simulink model "main_ddp_N5"  (R2026a)
settings: Solver=VariableStepAuto  StopTime=simulation_time  FixedStep=params.MPC.dt  RelTol=1e-2
undefined symbols (not defined in the file or in its folder): params, Ref
(part 1 of 2)
settings Model: Creator=katsu  LastModifiedBy=hoshino

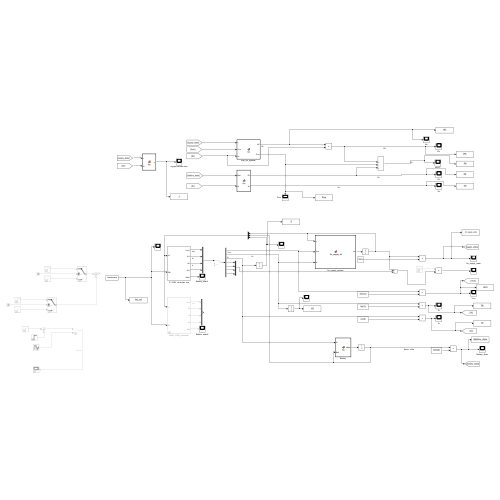
[thumbnail: Simulink's stored preview of the top-level diagram]
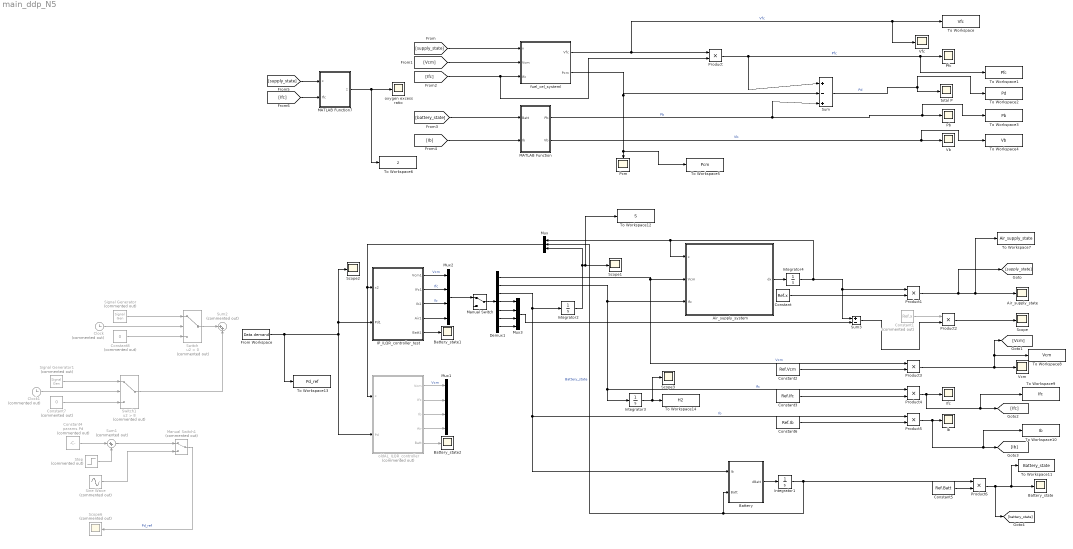
== system main_ddp_N5 ==
  Air_supply_state : Scope
      settings: ActiveDisplayYMinimum=-12592.967592784222  ActiveDisplayYMaximum=162770.79990525215  DataLoggingVariableName=ScopeData3
  Air_supply_system : MATLAB Function  TreatAsAtomicUnit=on
  Battery : MATLAB Function  TreatAsAtomicUnit=on
  Battery_state : Scope
      settings: ActiveDisplayYMinimum=-1  ActiveDisplayYMaximum=1  DataLoggingVariableName=ScopeData2
  Battery_state1 : Scope
      settings: ActiveDisplayYMinimum=-0.0625  ActiveDisplayYMaximum=0.5625
  Battery_state2 : Scope
      settings: ActiveDisplayYMinimum=-0.0625  ActiveDisplayYMaximum=0.5625
  Clock : Clock  Commented=on
  Clock1 : Clock  Commented=on
  Constant : Constant  Value=Ref.x
  Constant1 : Constant  Commented=on  Value=Ref.x
  Constant2 : Constant  Value=Ref.Vcm
  Constant3 : Constant  Value=Ref.Ifc
  Constant4 : Constant  Commented=on  Value=params.Pd
  Constant5 : Constant  Value=Ref.Batt
  Constant6 : Constant  Value=Ref.Ib
  Constant7 : Constant  Commented=on  Value=0
  Constant8 : Constant  Commented=on  Value=0
  Demux1 : Demux  Outputs=7
  From Workspace : FromWorkspace  VariableName=Data.demand
  IP_ILQR_controller_test : Subsystem
  Ib : Scope
      settings: ActiveDisplayYMinimum=-4.4974516854867295  ActiveDisplayYMaximum=40.486661709078128  DataLoggingVariableName=ScopeData3
  Ifc : Scope
      settings: ActiveDisplayYMinimum=31.92108  ActiveDisplayYMaximum=418.48985  DataLoggingVariableName=ScopeData2
  Integrator1 : Integrator  InitialCondition=params.start.Bat./Ref.Batt
  Integrator2 : Integrator
  Integrator3 : Integrator
  Integrator4 : Integrator  InitialCondition=params.start.x ./[Ref.x]
  MATLAB Function : MATLAB Function  TreatAsAtomicUnit=on
  MATLAB Function7 : MATLAB Function  TreatAsAtomicUnit=on
  Manual Switch : ManualSwitch
  Manual Switch1 : ManualSwitch  Commented=on
  Mux : Mux  Inputs=3
  Mux1 : Mux
  Mux2 : Mux
  Mux3 : Mux
  Pb : Scope
      settings: ActiveDisplayYMinimum=-1  ActiveDisplayYMaximum=1  DataLoggingVariableName=ScopeData6
  Pcm : Scope
      settings: ActiveDisplayYMinimum=1718.35704  ActiveDisplayYMaximum=9747.00989  DataLoggingVariableName=ScopeData4
  Pfc : Scope
      settings: ActiveDisplayYMinimum=-1238.1930512276633  ActiveDisplayYMaximum=24168.684595902479  DataLoggingVariableName=ScopeData5
  Product{,1..6} (7 alike) : Product
  Scope{,1..3} (4 alike) : Scope
      Scope settings: ActiveDisplayYMinimum=-1  ActiveDisplayYMaximum=1  DataLoggingVariableName=ScopeData3
      Scope1 settings: ActiveDisplayYMinimum=-0.37216  ActiveDisplayYMaximum=2.27993
      Scope2 settings: ActiveDisplayYMinimum=20919.76712  ActiveDisplayYMaximum=45919.76712
      Scope3 settings: ActiveDisplayYMinimum=-0.23032  ActiveDisplayYMaximum=2.07287
  Scope6 : Scope  Commented=on
      settings: ActiveDisplayYMinimum=23419.76712  ActiveDisplayYMaximum=33419.76712
  Signal Generator : SignalGenerator  Commented=on  WaveForm=square  Amplitude=10000  Frequency=0.5  Units=rad/sec
  Signal Generator1 : SignalGenerator  Commented=on  WaveForm=square  Amplitude=10000  Frequency=0.8  Units=rad/sec
  Sine Wave : Sin  Commented=on  Amplitude=1000  Bias=params.Pd  SampleTime=0
  Step : Step  Commented=on  FinalValue=10000  SampleTime=0
  Sum : Sum  Inputs=|+-+
  Sum1 : Sum  Commented=on  Inputs=|++
  Sum2 : Sum  Commented=on  Inputs=|++
  Sum3 : Sum  Inputs=+-
  Switch : Switch  Commented=on  Criteria=u2 > Threshold  SaturateOnIntegerOverflow=off  InputSameDT=off
  Switch1 : Switch  Commented=on  Criteria=u2 > Threshold  Threshold=8  SaturateOnIntegerOverflow=off  InputSameDT=off
  To Workspace : ToWorkspace  VariableName=Vfc  SaveFormat=Timeseries  SampleTime=-1
  To Workspace1 : ToWorkspace  VariableName=Pfc  SaveFormat=Timeseries  SampleTime=-1
  To Workspace10 : ToWorkspace  VariableName=Ib  SaveFormat=Timeseries  SampleTime=-1
  To Workspace11 : ToWorkspace  VariableName=Battery_state  SaveFormat=Timeseries  SampleTime=-1
  To Workspace12 : ToWorkspace  VariableName=S  SaveFormat=Timeseries  SampleTime=-1
  To Workspace13 : ToWorkspace  VariableName=Pd_ref  SaveFormat=Timeseries  SampleTime=-1
  To Workspace14 : ToWorkspace  VariableName=H2  SaveFormat=Timeseries  SampleTime=-1
  To Workspace2 : ToWorkspace  VariableName=Pd  SaveFormat=Timeseries  SampleTime=-1
  To Workspace3 : ToWorkspace  VariableName=Pb  SaveFormat=Timeseries  SampleTime=-1
  To Workspace4 : ToWorkspace  VariableName=Vb  SaveFormat=Timeseries  SampleTime=-1
  To Workspace5 : ToWorkspace  VariableName=Pcm  SaveFormat=Timeseries  SampleTime=-1
  To Workspace6 : ToWorkspace  VariableName=z  SaveFormat=Timeseries  SampleTime=-1
  To Workspace7 : ToWorkspace  VariableName=Air_supply_state  SaveFormat=Timeseries  SampleTime=-1
  To Workspace8 : ToWorkspace  VariableName=Vcm  SaveFormat=Timeseries  SampleTime=-1
  To Workspace9 : ToWorkspace  VariableName=Ifc  SaveFormat=Timeseries  SampleTime=-1
  Vb : Scope
      settings: ActiveDisplayYMinimum=44.990004314745107  ActiveDisplayYMaximum=45.709559071754136
  Vcm : Scope
      settings: ActiveDisplayYMinimum=74.317686308456928  ActiveDisplayYMaximum=124.19339407653175  DataLoggingVariableName=ScopeData2
  Vfc : Scope
      settings: ActiveDisplayYMinimum=227.63486  ActiveDisplayYMaximum=271.61772
  fuel_cel_systeml : MATLAB Function  TreatAsAtomicUnit=on
  oldAL_ILQR_controller : Subsystem  Commented=on
  oxygen excess ratio : Scope
      settings: ActiveDisplayYMinimum=-0.60546746114503058  ActiveDisplayYMaximum=29.452407830989813  DataLoggingVariableName=ScopeData4
  total P : Scope
      settings: ActiveDisplayYMinimum=918.68387588159749  ActiveDisplayYMaximum=19809.090544344064
  wires:
  Battery/1(dBatt) -> Integrator1/1
  Integrator1/1 -> Product6/1, Battery/2(Batt), Mux/2  "Battery_state"
  Air_supply_system/1(dx) -> Integrator4/1
  Demux1/1 -> Product3/1, Air_supply_system/2(Vcm)  "Vcm"
  Integrator4/1 -> Air_supply_system/1(x), Mux/1, Product1/1, Sum3/1
  MATLAB Function7/1(z) -> To Workspace6/1, oxygen excess ratio/1
  Demux1/2 -> Integrator3/1, Product4/1, Air_supply_system/3(Ifc)  "Ifc"
  Mux/1 -> oldAL_ILQR_controller/1(x), IP_ILQR_controller_test/1(x2)
  Demux1/3 -> Product5/1, Battery/1(Ib), Integrator2/1  "Ib"
  Sum/1 -> To Workspace2/1, total P/1  "Pd"
  Product/1 -> Sum/1, To Workspace1/1, Pfc/1  "Pfc"
  MATLAB Function/1(Pb) -> To Workspace3/1, Pb/1, Sum/3  "Pb"
  fuel_cel_systeml/1(Vfc) -> Vfc/1, To Workspace/1, Product/1  "Vfc"
  fuel_cel_systeml/2(Pcm) -> Sum/2, To Workspace5/1, Pcm/1
  MATLAB Function/2(Vb) -> To Workspace4/1, Vb/1  "Vb"
  Manual Switch1/1 -> Scope6/1  "Pd_ref"
  Mux3/1 -> Sum3/2
  Product1/1 -> [supply_state], To Workspace7/1, Air_supply_state/1
  Constant/1 -> Product1/2
  Constant1/1 -> Product2/1
  Sum3/1 -> Product2/2
  Product2/1 -> Scope/1
  Product3/1 -> To Workspace8/1, [Vcm], Vcm/1
  Product5/1 -> To Workspace10/1, [Ib], Ib/1
  Constant3/1 -> Product4/2
  Constant2/1 -> Product3/2
  Constant6/1 -> Product5/2
  Product4/1 -> To Workspace9/1, [Ifc], Ifc/1
  [Ifc] -> Product/2, fuel_cel_systeml/3(Ifc)
  [Vcm] -> fuel_cel_systeml/2(Vcm)
  [supply_state] -> fuel_cel_systeml/1(x)
  [Ib] -> MATLAB Function/2(Ib)
  [battery_state] -> MATLAB Function/1(Batt)
  [supply_state] -> MATLAB Function7/1(x)
  [Ifc] -> MATLAB Function7/2(Ifc)
  Constant5/1 -> Product6/2
  IP_ILQR_controller_test/5(Batt1) -> Battery_state1/1
  Integrator2/1 -> To Workspace12/1, Scope1/1, Mux/3
  Sine Wave/1 -> Manual Switch1/2
  Constant4/1 -> Sum1/1
  Clock/1 -> Switch/2
  Constant8/1 -> Switch/3
  Signal Generator/1 -> Switch/1
  Signal Generator1/1 -> Switch1/1
  Constant7/1 -> Switch1/3
  Switch1/1 -> Sum2/2
  Clock1/1 -> Switch1/2
  Switch/1 -> Sum2/1
  Product6/1 -> [battery_state], To Workspace11/1, Battery_state/1
  Sum1/1 -> Manual Switch1/1
  Step/1 -> Sum1/2
  From Workspace/1 -> Scope2/1, IP_ILQR_controller_test/2(Pd1), oldAL_ILQR_controller/2(Pd), To Workspace13/1
  Integrator3/1 -> Scope3/1, To Workspace14/1
  oldAL_ILQR_controller/5(Batt) -> Battery_state2/1
  oldAL_ILQR_controller/3(Ib) -> Mux1/3
  oldAL_ILQR_controller/2(Ifc) -> Mux1/2
  oldAL_ILQR_controller/1(Vcm) -> Mux1/1  "Vcm"
  oldAL_ILQR_controller/4(Air) -> Mux1/4
  IP_ILQR_controller_test/2(Ifc1) -> Mux2/2  "Ifc"
  IP_ILQR_controller_test/1(Vcm1) -> Mux2/1  "Vcm"
  IP_ILQR_controller_test/3(Ib1) -> Mux2/3  "Ib"
  IP_ILQR_controller_test/4(Air1) -> Mux2/4
  Mux2/1 -> Manual Switch/1
  Demux1/4 -> Mux3/1
  Demux1/5 -> Mux3/2
  Demux1/6 -> Mux3/3
  Demux1/7 -> Mux3/4
  Manual Switch/1 -> Demux1/1

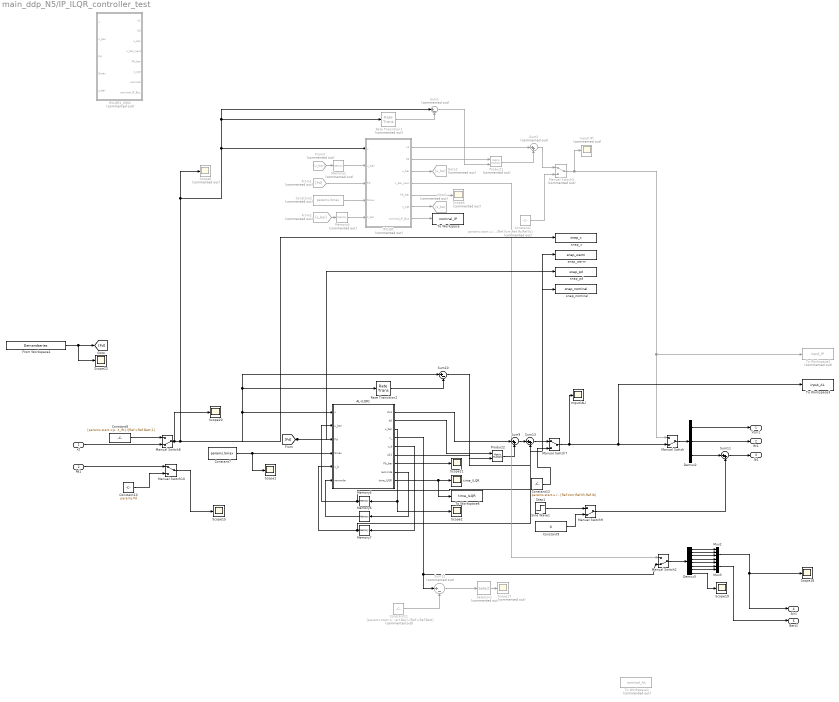
== system main_ddp_N5/IP_ILQR_controller_test ==
  x2 : Inport
  Pd1 : Inport  Port=2
  AL-ILQR1 : MATLAB Function  TreatAsAtomicUnit=on  SystemSampleTime=params.MPC.dt
  Constant1 : Constant  Commented=on  Value=params.start.u./[Ref.Vcm;Ref.Ifc;Ref.Ib]
  Constant10 : Constant  Value=params.Pd
  Constant11 : Constant  Commented=on  Value=[params.start.x;params.start.Bat]./[Ref.x;Ref.Batt]
  Constant12 : Constant  Value=params.start.u./[Ref.Vcm;Ref.Ifc;Ref.Ib]
  Constant2 : Constant  Commented=on  Value=params.Smax
  Constant6 : Constant  Value=[params.start.x;params.start.Bat;params.start.int_Ifc]./[Ref.x;Ref.Batt;1]
  Constant7 : Constant  Value=params.Smax
  Constant9 : Constant  Value=0
  Demux2 : Demux  Outputs=3
  Demux3 : Demux  Outputs=8
  From Workspace1 : FromWorkspace  VariableName=Demandseries
  From1 : From  Commented=on  GotoTag=Pd
  From2 : From  Commented=on  GotoTag=s_bar
  From3 : From  Commented=on  GotoTag=u_bar
  Goto1 : Goto  Commented=on  GotoTag=s_bar
  Goto2 : Goto  Commented=on  GotoTag=u_bar
  IP-ILQR : MATLAB Function  Commented=on  TreatAsAtomicUnit=on  SystemSampleTime=params.MPC.dt
  IP-ILQR1_0902 : MATLAB Function  Commented=on  TreatAsAtomicUnit=on  SystemSampleTime=params.MPC.dt
  Imput(AL) : Scope
      settings: ActiveDisplayYMinimum=-0.12487486883862278  ActiveDisplayYMaximum=1.1244066421547534  DataLoggingVariableName=input_AL
  Input(IP) : Scope  Commented=on
      settings: TimeSpan=5  ActiveDisplayYMinimum=-0.2  ActiveDisplayYMaximum=1.2  DataLoggingVariableName=input_IP
  Manual Switch{,2,8..9} (4 alike) : ManualSwitch  CurrentSetting=0
  Manual Switch10 : ManualSwitch
  Manual Switch3 : ManualSwitch  Commented=on
  Manual Switch7 : ManualSwitch
  Memory1 : Memory  Commented=on  InitialCondition=repmat(params.start.u ,1,params.MPC.N)./[Ref.Vcm;Ref.Ifc;Ref.Ib]  InheritSampleTime=on  LinearizeAsDelay=on
  Memory4 : Memory  Commented=on  InitialCondition=params.start.s  InheritSampleTime=on  LinearizeAsDelay=on
  Memory5 : Memory  InitialCondition=repmat(params.start.u ,1,params.MPC.N)./[Ref.Vcm;Ref.Ifc;Ref.Ib]  InheritSampleTime=on  LinearizeAsDelay=on
  Memory6 : Memory  InitialCondition=zeros(params.nc,params.MPC.N+1)  InheritSampleTime=on  LinearizeAsDelay=on
  Memory7 : Memory  InitialCondition=repmat(params.start.u ,1,params.MPC.N)./[Ref.Vcm;Ref.Ifc;Ref.Ib]  InheritSampleTime=on  LinearizeAsDelay=on
  Mux2 : Mux
  Mux3 : Mux  Inputs=3
  Product1 : Product  Commented=on  Multiplication=Matrix(*)
  Product2 : Product  Multiplication=Matrix(*)
  Rate Transition1 : RateTransition  Commented=on  OutPortSampleTime=params.MPC.dt
  Rate Transition2 : RateTransition  OutPortSampleTime=params.MPC.dt
  Scope{1..2,15,18..22} (8 alike) : Scope
      Scope1 settings: ActiveDisplayYMinimum=-1  ActiveDisplayYMaximum=1
      Scope15 settings: ActiveDisplayYMinimum=22667.97504  ActiveDisplayYMaximum=30185.8959  DataLoggingVariableName=ScopeData11
      Scope18 settings: ActiveDisplayYMinimum=-0.12272  ActiveDisplayYMaximum=1.39941  DataLoggingVariableName=ScopeData14
      Scope19 settings: ActiveDisplayYMinimum=-0.01265  ActiveDisplayYMaximum=0.11382  DataLoggingVariableName=ScopeData15
      Scope2 settings: ActiveDisplayYMinimum=-0.12443232387072894  ActiveDisplayYMaximum=1.1249110476521393  DataLoggingVariableName=ScopeData7
      Scope20 settings: ActiveDisplayYMinimum=-0.15593  ActiveDisplayYMaximum=1.40334  DataLoggingVariableName=ScopeData16
      Scope21 settings: ActiveDisplayYMinimum=-194.73385  ActiveDisplayYMaximum=1761.44655  DataLoggingVariableName=ScopeData17
      Scope22 settings: ActiveDisplayYMinimum=-1  ActiveDisplayYMaximum=1
  Scope17 : Scope  Commented=on
      settings: ActiveDisplayYMinimum=-344.77426  ActiveDisplayYMaximum=3043.62299  DataLoggingVariableName=ScopeData13
  Scope4 : Scope  Commented=on
      settings: ActiveDisplayYMinimum=-2111.11617  ActiveDisplayYMaximum=1957.87921  DataLoggingVariableName=ScopeData2
  Scope6 : Scope  Commented=on
      settings: ActiveDisplayYMinimum=-0.37396  ActiveDisplayYMaximum=3.36567
  Selector1 : Selector  Commented=on  InputPortWidth=7  IndexOptions=Index vector (dialog)  Indices=[1:4 1]  OutputSizes=1
  Sine Wave1 : Sin  Amplitude=10/Ref.Ib  SampleTime=0
  Step1 : Step  Time=3  InitialValue=-10  FinalValue=10  SampleTime=0
  Sum1 : Sum  Commented=on  Inputs=|+-
  Sum10 : Sum  Inputs=|+-
  Sum11 : Sum  Inputs=|++
  Sum12 : Sum  Commented=on  Inputs=|+-
  Sum13 : Sum  Inputs=|++
  Sum2 : Sum  Commented=on  Inputs=|++
  Sum9 : Sum  Inputs=|++
  To Workspace : ToWorkspace  VariableName=nominal_IP  SaveFormat=Timeseries  SampleTime=-1
  To Workspace1 : ToWorkspace  Commented=on  VariableName=nominal_AL  SaveFormat=Timeseries  SampleTime=-1
  To Workspace2 : ToWorkspace  Commented=on  VariableName=input_IP  SaveFormat=Timeseries  SampleTime=-1
  To Workspace3 : ToWorkspace  VariableName=input_AL  SaveFormat=Timeseries  SampleTime=-1
  To Workspace6 : ToWorkspace  VariableName=time_ILQR  SaveFormat=Timeseries  SampleTime=-1
  snap_nominal : ToWorkspace  VariableName=snap_nominal  SaveFormat=Timeseries  SampleTime=params.MPC.dt
  snap_pd : ToWorkspace  VariableName=snap_pd  SaveFormat=Timeseries  SampleTime=params.MPC.dt
  snap_warm : ToWorkspace  VariableName=snap_warm  SaveFormat=Timeseries  SampleTime=params.MPC.dt
  snap_x : ToWorkspace  VariableName=snap_x  SaveFormat=Timeseries  SampleTime=params.MPC.dt
  time_ILQR : Scope
      settings: ActiveDisplayYMinimum=0.077124575000000015  ActiveDisplayYMaximum=0.41982182499999993  DataLoggingVariableName=ScopeData8
  Vcm1 : Outport
  Ifc1 : Outport  Port=2
  Ib1 : Outport  Port=3
  Air1 : Outport  Port=4
  Batt1 : Outport  Port=5
  wires:
  Manual Switch3/1 -> To Workspace2/1, Manual Switch/1, Input(IP)/1
  Constant11/1 -> Sum12/2
  AL-ILQR1/6(ub1) -> Sum13/2
  Sum10/1 -> Product2/2
  AL-ILQR1/5(u_b) -> Memory7/1
  AL-ILQR1/3(u_bar) -> Scope2/1, Memory5/1
  Sine Wave1/1 -> Manual Switch9/1
  Demux3/2 -> Mux2/2
  Demux3/5 -> Mux3/1
  Memory7/1 -> AL-ILQR1/5("u_b "), snap_nominal/1
  AL-ILQR1/2(K0) -> Product2/1
  Constant9/1 -> Manual Switch9/2
  Memory6/1 -> AL-ILQR1/6("rammda ")
  Constant7/1 -> Scope1/1, AL-ILQR1/4(Smax)
  Sum13/1 -> Manual Switch7/1
  AL-ILQR1/4(x_) -> Manual Switch2/2, Sum12/1
  Constant12/1 -> Manual Switch7/2
  Demux3/8 -> Scope19/1
  AL-ILQR1/8(rammda) -> Memory6/1
  Demux3/3 -> Mux2/3
  Sum11/1 -> Ib1/1
  Sum9/1 -> Sum13/1
  Demux3/4 -> Mux2/4
  Demux2/1 -> Vcm1/1
  Pd1/1 -> Manual Switch10/1
  AL-ILQR1/1(du1) -> Sum9/1
  Memory5/1 -> AL-ILQR1/2("u_bar "), snap_warm/1
  Constant6/1 -> Manual Switch8/1
  Demux3/7 -> Mux3/3
  Mux2/1 -> Scope18/1, Air1/1
  Demux2/2 -> Ifc1/1
  Demux3/1 -> Mux2/1
  Demux3/6 -> Mux3/2
  Selector1/1 -> Scope17/1
  Constant10/1 -> Manual Switch10/2
  Product2/1 -> Sum9/2
  Manual Switch7/1 -> To Workspace3/1, Manual Switch/2, Imput(AL)/1
  x2/1 -> Manual Switch8/2
  Manual Switch10/1 -> Scope15/1
  Rate Transition2/1 -> Sum10/2
  Mux3/1 -> Batt1/1
  Demux2/3 -> Sum11/1
  AL-ILQR1/7(Pb_bar) -> Scope21/1
  Sum12/1 -> Selector1/1
  Manual Switch9/1 -> Sum11/2
  Manual Switch/1 -> Demux2/1
  Manual Switch2/1 -> Demux3/1
  IP-ILQR/4(x_bar_next) -> Manual Switch2/1
  Constant1/1 -> Manual Switch3/2
  Sum1/1 -> Product1/2
  IP-ILQR/5(Pb_bar) -> Scope4/1
  Constant2/1 -> IP-ILQR/4(Smax)
  Memory1/1 -> IP-ILQR/2("u_bar ")
  IP-ILQR/2(K0) -> Product1/1
  Sum2/1 -> Manual Switch3/1
  Rate Transition1/1 -> Sum1/2
  Product1/1 -> Sum2/2
  Manual Switch8/1 -> Scope20/1, Scope6/1, Sum1/1, Rate Transition1/1, IP-ILQR/1(x), Sum10/1, Rate Transition2/1, AL-ILQR1/1(x), snap_x/1
  From1/1 -> IP-ILQR/3(Pd)
  [Pd] -> AL-ILQR1/3(Pd), snap_pd/1
  From Workspace1/1 -> Scope22/1, [Pd]
  Memory4/1 -> IP-ILQR/5(s_bar)
  IP-ILQR/1(u1) -> Sum2/1
  IP-ILQR/7(nominal_IP_Bus) -> To Workspace/1
  ? -> To Workspace1/1
  IP-ILQR/6(s_opt) -> Goto1/1
  From2/1 -> Memory4/1
  IP-ILQR/3(u_bar) -> Goto2/1
  From3/1 -> Memory1/1
  AL-ILQR1/9(time_ILQR) -> To Workspace6/1, time_ILQR/1

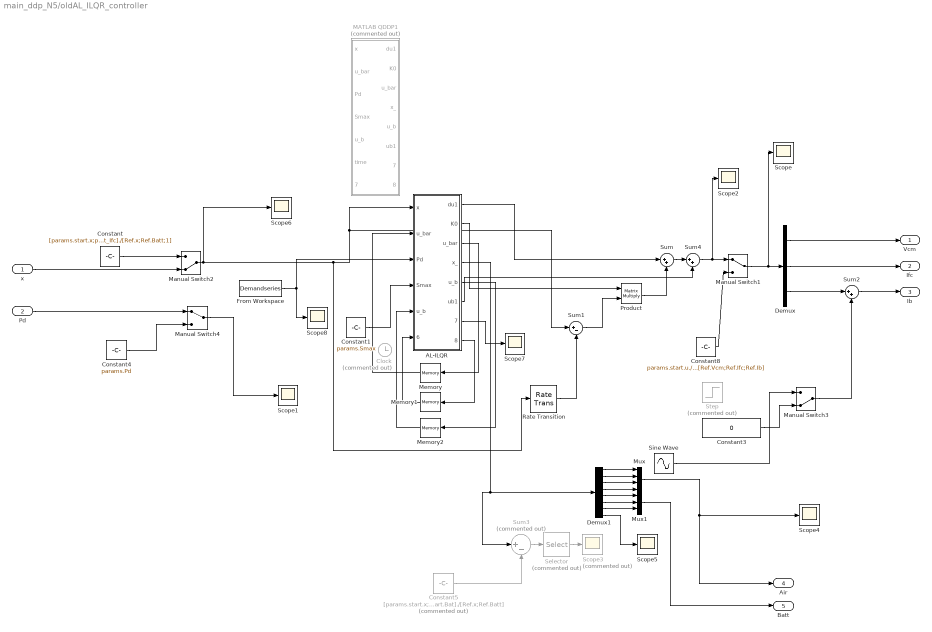
== system main_ddp_N5/oldAL_ILQR_controller ==
  x : Inport
  Pd : Inport  Port=2
  AL-ILQR : MATLAB Function  TreatAsAtomicUnit=on  SystemSampleTime=params.MPC.dt
  Clock : Clock  Commented=on
  Constant : Constant  Value=[params.start.x;params.start.Bat;params.start.int_Ifc]./[Ref.x;Ref.Batt;1]
  Constant1 : Constant  Value=params.Smax
  Constant3 : Constant  Value=0
  Constant4 : Constant  Value=params.Pd
  Constant5 : Constant  Commented=on  Value=[params.start.x;params.start.Bat]./[Ref.x;Ref.Batt]
  Constant8 : Constant  Value=params.start.u./[Ref.Vcm;Ref.Ifc;Ref.Ib]
  Demux : Demux  Outputs=3
  Demux1 : Demux  Outputs=8
  From Workspace : FromWorkspace  VariableName=Demandseries
  MATLAB QDDP1 : MATLAB Function  Commented=on  TreatAsAtomicUnit=on  SystemSampleTime=params.MPC.dt
  Manual Switch1 : ManualSwitch
  Manual Switch2 : ManualSwitch  CurrentSetting=0
  Manual Switch3 : ManualSwitch  CurrentSetting=0
  Manual Switch4 : ManualSwitch
  Memory : Memory  InitialCondition=repmat(params.start.u ,1,params.MPC.N)./[Ref.Vcm;Ref.Ifc;Ref.Ib]  InheritSampleTime=on  LinearizeAsDelay=on
  Memory1 : Memory  InitialCondition=zeros(params.nc,params.MPC.N+1)  InheritSampleTime=on  LinearizeAsDelay=on
  Memory2 : Memory  InitialCondition=repmat(params.start.u ,1,params.MPC.N)./[Ref.Vcm;Ref.Ifc;Ref.Ib]  InheritSampleTime=on  LinearizeAsDelay=on
  Mux : Mux
  Mux1 : Mux  Inputs=3
  Product : Product  Multiplication=Matrix(*)
  Rate Transition : RateTransition  OutPortSampleTime=params.MPC.dt
  Scope{,1..2,4..8} (8 alike) : Scope
      Scope settings: ActiveDisplayYMinimum=-0.39118  ActiveDisplayYMaximum=0.89561  DataLoggingVariableName=ScopeData3
      Scope1 settings: ActiveDisplayYMinimum=22667.97504  ActiveDisplayYMaximum=30185.8959  DataLoggingVariableName=ScopeData4
      Scope2 settings: ActiveDisplayYMinimum=-0.04167  ActiveDisplayYMaximum=0.375
      Scope4 settings: ActiveDisplayYMinimum=-0.10905  ActiveDisplayYMaximum=1.47496
      Scope5 settings: ActiveDisplayYMinimum=-0.01265  ActiveDisplayYMaximum=0.11382  DataLoggingVariableName=ScopeData2
      Scope6 settings: ActiveDisplayYMinimum=-0.23275  ActiveDisplayYMaximum=2.09474
      Scope7 settings: ActiveDisplayYMinimum=-152.32904  ActiveDisplayYMaximum=1463.33798
      Scope8 settings: ActiveDisplayYMinimum=20919.76712  ActiveDisplayYMaximum=45919.76712  DataLoggingVariableName=ScopeData2
  Scope3 : Scope  Commented=on
      settings: ActiveDisplayYMinimum=-344.77426  ActiveDisplayYMaximum=3043.62299  DataLoggingVariableName=ScopeData2
  Selector : Selector  Commented=on  InputPortWidth=7  IndexOptions=Index vector (dialog)  Indices=[1:4 1]  OutputSizes=1
  Sine Wave : Sin  Amplitude=10/Ref.Ib  SampleTime=0
  Step : Step  Commented=on  Time=3  InitialValue=-10  FinalValue=10  SampleTime=0
  Sum : Sum  Inputs=|++
  Sum1 : Sum  Inputs=|+-
  Sum2 : Sum  Inputs=|++
  Sum3 : Sum  Commented=on  Inputs=|+-
  Sum4 : Sum  Inputs=|++
  Vcm : Outport
  Ifc : Outport  Port=2
  Ib : Outport  Port=3
  Air : Outport  Port=4
  Batt : Outport  Port=5
  wires:
  Rate Transition/1 -> Sum1/2
  AL-ILQR/1(du1) -> Sum/1
  Sum1/1 -> Product/2
  Product/1 -> Sum/2
  AL-ILQR/2(K0) -> Product/1
  Memory/1 -> AL-ILQR/2("u_bar ")
  AL-ILQR/3(u_bar) -> Memory/1
  Demux/1 -> Vcm/1
  Demux/2 -> Ifc/1
  Constant8/1 -> Manual Switch1/2
  Manual Switch1/1 -> Scope/1, Demux/1
  AL-ILQR/4(x_) -> Sum3/1, Demux1/1
  x/1 -> Manual Switch2/2
  Constant/1 -> Manual Switch2/1
  Sum2/1 -> Ib/1
  Demux/3 -> Sum2/1
  Manual Switch3/1 -> Sum2/2
  Constant3/1 -> Manual Switch3/2
  Sine Wave/1 -> Manual Switch3/1
  Pd/1 -> Manual Switch4/1
  Manual Switch4/1 -> Scope1/1
  Constant4/1 -> Manual Switch4/2
  Selector/1 -> Scope3/1
  Sum3/1 -> Selector/1
  Constant5/1 -> Sum3/2
  Mux/1 -> Scope4/1, Air/1
  Demux1/1 -> Mux/1
  Demux1/2 -> Mux/2
  Demux1/3 -> Mux/3
  Demux1/4 -> Mux/4
  Demux1/5 -> Mux1/1
  Demux1/6 -> Mux1/2
  Demux1/7 -> Mux1/3
  Mux1/1 -> Batt/1
  Manual Switch2/1 -> Scope6/1, Rate Transition/1, AL-ILQR/1(x), Sum1/1
  Demux1/8 -> Scope5/1
  Constant1/1 -> AL-ILQR/4(Smax)
  AL-ILQR/5(u_b) -> Memory2/1
  Memory2/1 -> AL-ILQR/5("u_b ")
  Sum/1 -> Sum4/1
  Sum4/1 -> Scope2/1, Manual Switch1/1
  AL-ILQR/6(ub1) -> Sum4/2
  AL-ILQR/7(Pb_bar) -> Scope7/1
  From Workspace/1 -> AL-ILQR/3(Pd), Scope8/1
  AL-ILQR/8(rammda) -> Memory1/1
  Memory1/1 -> AL-ILQR/6("rammda ")

== matlab function main_ddp_N5/oldAL_ILQR_controller/AL-ILQR ==
  data: x input size=params.nx; u_bar input size=[params.nu,params.MPC.N]; du1 output size=params.nu; Pd input; K0 output size=[params.nu,params.nx]; u_bar output size=[params.nu,params.MPC.N]; params parameter; x_ output size=params.nx; Ref parameter; Smax input; u_b input; u_b output; ub1 output size=[params.nu 1]; Pb_bar output size=1; rammda input; rammda output
function [du1,K0,u_bar,x_,u_b,ub1,Pb_bar,rammda] = ILQR(x,u_bar,Pd,params,Ref,Smax,u_b,rammda)
%UNTITLED3 この関数の概要をここに記述
%   詳細説明をここに記述
du = u_bar-u_b;
% which discretization method
D_method = 'V';                 % D:difference, V:variational


%%%%%%%%%%%%%%%%%%%%%% MPC setting %%%%%%%%%%%%%%%%%%%%%%%%%%%%%%%%%%%%%%%%
% linesearch off:0 on:1
linesearch = 1;
tsp = params.MPC.dt;            % sampling period
N = 10;                         % number of horizon 
N_iter = params.N_iter;         % number of N_iter


nx = size(x,1);                 
nu = size(u_bar,1);             
K0 = zeros(nu,nx);             
x_bar = zeros(nx,N+1);

%%%%%%%%%%%%%%%%% Augumented Lagrangian setting %%%%%%%%%%%%%%%%%%%%%%%%%%%
nc = 15 ;
nc_i = params.nc_i;
Altro.mu = repmat(4e-4,nc,N+1);
Altro.I_mu = zeros(nc,(N+1)*nc);
Altro.rammda = rammda;
Altro.rammda = zeros(nc,N+1);
Altro.cmax = 1e-8;
Altro.phi = 2;
Value_c = ones(nc,N+1);

for i = 1:N_iter

     for ii = 1:N+1
         for jj = 1:nc
                if Value_c(jj,ii) < 0 && Altro.rammda(jj,ii) == 0 && jj <= nc_i
                    Altro.I_mu(jj,nc*(ii-1)+jj) = 0;
                else
                    Altro.I_mu(jj,nc*(ii-1)+jj) = Altro.mu(jj,ii);
                if Altro.mu(jj,ii)<=100
                    Altro.mu(jj,ii) = Altro.mu(jj,ii)*Altro.phi;
                end
                end

         end
    end

          disp(i)
          disp('--------------')


    [x_bar,A,B] = forwardpass(x,u_b,du,tsp,N,D_method,params,Ref);
    [du,K0] = backwardpass_Altro_e(x_bar,u_b,du,A,B,N,tsp,linesearch,Pd,params,Altro,Ref,Smax,u_b);
    % [x_bar,A,B] = forwardpass_runge(x,u_b,du,tsp,N,D_method,params,Ref);
    % [du,K0] = backwardpass_Altro_e_runge(x_bar,u_b,du,A,B,N,tsp,linesearch,Pd,params,Altro,Ref,Smax);
        for ii = 1:N+1

            if ii ~= N+1
                [x_bar(:,ii),du(:,ii)] = satulation(x_bar(:,ii),u_b(:,ii),du(:,ii));
                if (x_bar(1,:)/0.1173+params.psat/Ref.pres) < 2
                    Value_c(:,ii) = constraints_case1(x_bar(:,ii),u_b(:,ii),du(:,ii),Pd(ii),Smax);
                else
                    Value_c(:,ii) = constraints_case2(x_bar(:,ii),u_b(:,ii),du(:,ii),Pd(ii),Smax);
                end
            else
                [x_bar(:,ii),~] = satulation(x_bar(:,ii),u_b(:,ii-1),du(:,ii-1));
                if (x_bar(1,:)/0.1173+params.psat/Ref.pres) < 2
                    Value_c(:,ii) = constraints_case1(x_bar(:,ii),u_b(:,ii-1),du(:,ii-1),Pd(ii-1),Smax);
                else
                    Value_c(:,ii) = constraints_case2(x_bar(:,ii),u_b(:,ii-1),du(:,ii-1),Pd(ii-1),Smax);
                end
            end

            for jj = 1:nc

                if Value_c(jj,ii) < 0 && Altro.rammda(jj,ii) == 0 && jj <= nc_i
                    Altro.rammda(jj,ii) = max([Altro.rammda(jj,ii) + Altro.mu(jj,ii).*Value_c(jj,ii),0]);
                elseif jj>nc_i
                    Altro.rammda(jj,ii) = Altro.rammda(jj,ii) + Altro.mu(jj,ii).*Value_c(jj,ii);
                else
                end

            end
            % disp(Altro.rammda(:,ii))
        end
end
rammda = circshift(Altro.rammda,-1,2);
rammda(:,end) = rammda(:,end-1);
ub1 = u_b(:,1);
u_bar = u_b+du;
Pb_bar = Pb_fun(x_bar(:,1),u_b(:,1),du(:,1));
x_ = x_bar(:,2);
du1 = du(:,1);
u_b = u_bar;
u_bar = circshift(u_b,-1,2);

u_bar(:,end) = u_b(:,end-1);

== matlab function main_ddp_N5/Air_supply_system ==
  data: x input; Vcm input; dx output size=4; Ifc input; params parameter; Ref parameter
function dx = Air_supply_4d(x,Vcm,Ifc,params,Ref)
%saturation
% if Vcm < 0  
%    Vcm = 150;
% elseif Vcm > params.Vcm_u/Ref.Vcm 
%    Vcm = params.Vcm_u/Ref.Vcm ;
% end
% 
% if Ifc < 0 
%     Ifc = 0;
% elseif Ifc > 2.2*params.Afc/Ref.Ifc   
%     Ifc = 2.2*params.Afc/Ref.Ifc;
% end

if params.c11/(x(1)+x(2)+params.c2/Ref.pres)>params.c19*Ref.pres
    dx = Air_supply_case1(x,[Vcm;Ifc],[0;0]);
else
    dx = Air_supply_case2(x,[Vcm;Ifc],[0;0]);
end

% x = x./[Ref.x];
% Vcm = Vcm./Ref.Vcm;
% Ifc = Ifc./Ref.Ifc;
% dx = dx.*[Ref.x];

% R_= 8.314;  %Universal gas constant
% patm = 1.01325e5;  %Atomospheric pressure
% psat = 4.736e4;  %Saturation pressure 353K 
% Tatm = 298.15;   %Atmosphric temperature
% Tst = 353.15;    %Temperature of fuel-cell stack 
% Mo2 = 32e-3; %Molar mass of oxygen
% Mn2 = 28e-3; %Molar mass of nitrogen
% Mv = 18.02e-3; %Molar mass of vapour
% Maatm = 28.97e-3; %Molar mass of atmospheric air
% gam = 1.4;  %Air specific heat ratio
% Cp = 1004;   %Air specific ratio
% F = 96487;  %Faraday's constant
% kt = 0.0153;    %motor constant
% kv = 0.0153;    %motor constant
% Rcm = 0.82;    %motor constant
% Jcp = 5e-5;     %compressor and motor interia
% eata_cp = 0.80; %Compressor efficiency
% eata_cm = 0.98; %Compressor motor mechanical efficiency
% n = 381;    %Number of cells in fuel-cell stack
% Afc = 280;   %Fuel-cell active area (cm^2)
% Vsm = 0.02;     %Supply manifold volume
% Vca = 0.01;     %Single stack cathode volume
% kcain = 0.3629e-5; %Cathode inlet orifice
% tm = 1.275e-4;
% Cd = 0.0124;    %Cathode output throttle discharge cofficient
% At = 0.002;     %Cathode output throttle area
% phi_atm = 0.5;  %Average ambient air relative humidity
% yo2atm = 0.21;  %Oxygen molar ratio at cathode inlet
% xo2atm =yo2atm*Mo2/(yo2atm*Mo2+(1-yo2atm)*Mn2); %Oxygen mass fraction at cathode inlet
% watm =Mv/(yo2atm*Mo2+(1-yo2atm)*Mn2)*(phi_atm*psat/(patm-phi_atm*psat)); %Humidity ratio of inlet air
% Kapper = sqrt(mean([Mo2^2,Mn2^2,Mv^2]));
% Vcm_u = 300;
% 
% c1 = (R_*Tst*kcain)/(Mo2*Vca)*(xo2atm/(1+watm));
% c2 = psat;
% c3 = R_*Tst/Vca;
% c4 = Mo2;
% c5 = Mn2;
% c6 = Mv*psat;
% c7 = (R_*Tst*n)/(4*Vca*F);
% c8 = (R_*Tst*kcain)/(Mn2*Vca)*((1-xo2atm)/(1+watm));
% c9 = eata_cm*kt*kv/(Jcp*Rcm);
% c10 = Cp*Tatm/(Jcp*eata_cp);
% c11 = patm;
% c12 = (gam-1/gam);
% c13 = eata_cm*kt/(Jcp*Rcm);
% c14 = R_*Tatm/(Maatm*Vsm);
% c15 = 1/eata_cp;
% c16 = kcain;
% c17 = (Cd*At)/sqrt(R_*Tst)*sqrt(2*gam/(gam-1));
% c18 = 1/gam;
% c19 = (2/(gam+1))^(gam/(gam-1));
% c20 = (Cd*At)/sqrt(R_*Tst)*gam^(1/2)*(2/(gam+1))^((gam+1)/2*(gam-1));
% c21 = 1/Rcm;
% c22 = kv;
% c23 = kcain*xo2atm/(1+watm);
% c24 = n*Mo2/(4*F);
% 
% 
% if c11/(x(1)+x(2)+c2) > c19
% dx = [
%     c1*(-x(1)-x(2)+x(4)-c2)-(c3*x(1)*psi_case1(x,c2,c11,c12,c17,c18,c19,c20))/(c4*x(1)+c5*x(2)+c6)-c7*Ifc;
%     c8*(-x(1)-x(2)+x(4)-c2)-(c3*x(2)*psi_case1(x,c2,c11,c12,c17,c18,c19,c20))/(c4*x(1)+c5*x(2)+c6);
%     -c9*x(3)-(c10./x(3))*((x(4)./c11).^c12-1)*Weight_flow(x(3),x(4))+c13*Vcm;
%     c14*(1+c15*((x(4)./c11)^c12-1))*(Weight_flow(x(3),x(4))-c16*(-x(1)-x(2)+x(4)-c2))];
% else
% 
% dx =  [
%     c1*(-x(1)-x(2)+x(4)-c2)-(c3*x(1)*psi_case2(x,c2,c11,c12,c17,c18,c19,c20))/(c4*x(1)+c5*x(2)+c6)-c7*Ifc;
%     c8*(-x(1)-x(2)+x(4)-c2)-(c3*x(2)*psi_case2(x,c2,c11,c12,c17,c18,c19,c20))/(c4*x(1)+c5*x(2)+c6);
%     -c9*x(3)-(c10./x(3))*((x(4)./c11).^c12-1)*Weight_flow(x(3),x(4))+c13*Vcm;
%     c14*(1+c15*((x(4)./c11)^c12-1))*(Weight_flow(x(3),x(4))-c16*(-x(1)-x(2)+x(4)-c2))];
% end
% 
% 
% 
% 
% %%%%%%%%%%%%%%%%%%%%%%%%%%%%%%%%%%%%%%%%%%%%%%%%%%%%%%%%%%%%%%%%%%%%%%%%%%%%
% 
% end
% 
% function psi = psi_case1(x,c2,c11,c12,c17,c18,c19,c20)
% psi = c17*(x(1)+x(2)+c2)*(c11/(x(1)+x(2)+c2))^c18*sqrt(1-(c11/(x(1)+x(2)+c2))^c12);
% end
% 
% function psi = psi_case2(x,c2,c11,c12,c17,c18,c19,c20)
% psi = c20*(x(1)+x(2)+c2);
% end

== matlab function main_ddp_N5/Battery ==
  data: Ib input; Batt input; dBatt output; Ref parameter; params parameter
function dBatt = fcn(Ib,Batt,Ref,params)
% if Ib <-36/Ref.Ib
%     Ib = -36/Ref.Ib;
% elseif Ib > 36/Ref.Ib
%     Ib = 36/Ref.Ib;
% end
% Ib = Ib/15; %pararel 15
% Battery() already converts pack current to cell current.

dBatt = Battery(Batt,Ib,0);
% Vsoc = Batt(1);
% Vs = Batt(2);
% Vf = Batt(3);

% Cb = 3060;
% SOC = Vsoc*100;
% Rsd = 10e9;
% Rs = 0.3208*exp(-29.14*SOC) +0.04669;
% Cs = -752.9*exp(-13.51*SOC) + 703.6;
% Rf = 6.603*exp(-155.2*SOC) +0.04984;
% Cf = -6056*exp(-27.12*SOC) + 4475;
% 
% 
% dVsoc = -Vsoc/(Rsd*Cb)-Ib/Cb;
% dVs = -Vs/(Rs*Cs)+Ib/Cs;
% dVf = -Vf/(Rf*Cf)+Ib/Cf;
% 
% dBatt = [dVsoc;dVs;dVf];

== matlab function main_ddp_N5/IP_ILQR_controller_test/IP-ILQR1_0902 ==
  data: x input size=params.nx; u_bar input size=[params.nu,params.MPC.N]; u1 output size=params.nu; Pd input; K0 output size=[params.nu,params.nx]; u_bar output size=[params.nu,params.MPC.N]; params parameter; x_bar_next output size=params.nx; Ref parameter; Smax input; Pb_bar output size=1; s_bar input; s_opt output; nominal output Bus: nominalBus; nominal_IP_Bus output Bus: nominal_IP_Bus
 function [u1,K0,u_bar, x_bar_next, Pb_bar, s_opt, nominal, nominal_IP_Bus] = ILQR(x,u_bar,Pd,params,Ref,Smax,s_bar)

% which discretization method
% D:difference, V:variational
D_method = 'D or V';
if params.D_method == 1
    D_method = 'D';       % 1:difference, 0:
    disp(D_method)
elseif params.D_method == 0
    D_method = 'V';
     % disp(D_method)
end

% 前の時間ステップからの時刻のずれを補正
u_bar(:,1:end-1) = u_bar(:,2:end);
u_bar(:,end)     = u_bar(:,end-1);
du = zeros(size(u_bar));

s_bar(:,1:end-1)   = s_bar(:,2:end);
s_bar(:,end)       = s_bar(:,end-1);

%%%%%%%%%%%%%%%%%%%%%% MPC setting %%%%%%%%%%%%%%%%%%%%%%%%%%%%%%%%%%%%%%%%
% linesearch off:0 on:1
linesearch = params.lineserch;
tsp = params.MPC.dt;            % sampling period
N = 10;                         % number of horizon 
N_iter = params.N_iter_IP;         % number of N_iter_IP

nx = size(x,1);                 
nu = size(u_bar,1);

K0 = zeros(nu,nx);             
x_bar = zeros(nx,N+1);
x_opt = zeros(nx,N+1);
du_IP = zeros(nu,N);
K0_IP = zeros(nu,nx);
x_opt_IP = zeros(nx,N+1);
du_opt = zeros(nu,N);



%%%%%%%%%%%%%%%%% Interior Point setting %%%%%%%%%%%%%%%%%%%%%%%%%%%%%%%%%
mu = params.MPC.mu;
mu_iter = params.mu_iter;
mu_decrease_rate = params.mu_decrease_rate;

disp('==========================0.05s')



s_opt = zeros(size(s_bar));
c    = zeros(size(s_bar));
c_mu = zeros(size(c,1),size(c,2),mu_iter);
r_mu = zeros(size(c_mu,1),size(c_mu,2),mu_iter);
s_mu = zeros(size(r_mu));
%%%%%%%%%%%%%%%%% Iteration %%%%%%%%%%%%%%%%%%%%%%%%%%%%%%%%%%%%%%%%%%%%%%%
ls_gamma = 1;

for j = 1:mu_iter
   for i = 1:N_iter
        % disp('--------------') 
        if any(x_bar(1,:) < 0)
           disp(u_bar+du)
           disp(x_bar)
        end
   
        [x_bar,A,B]    = forwardpass_runge(x, u_bar, du, tsp, N, D_method,params,Ref);
        [du_opt, x_opt,s_opt,K0,ls_gamma] = backwardpass_IP(x_bar, u_bar, du, s_bar,A,B,N,tsp,ls_gamma,Pd,params,mu,Ref,Smax);
        du = du_opt;

                     
   end
    % % % % % % % % % % % % % % % % % % % % % % % % % % % % % % % % % % % % % % % % % % % % % 
    %　各muでの r=s*c+muの計算
    for ii = 1:N
        if (x_opt(1,ii)/0.1173+params.psat/Ref.pres) < 2    
             c(:,ii) = constraints_case1(x_opt(:,ii),u_bar(:,ii),du_opt(:,ii),Pd(ii),Smax);
        else
             c(:,ii) = constraints_case2(x_opt(:,ii),u_bar(:,ii),du_opt(:,ii),Pd(ii),Smax);
        end
    end

    for ii = 1:N
        r_mu(:,ii,j)   = s_opt(:,ii).*c(:,ii)+mu;
        %r_mu(:,ii,j)   = s_opt(:,ii).*c(:,ii);
    end

    c_mu(:,:,j) = c;
    s_mu(:,:,j) = s_opt;
    disp(j)
    disp(mu')
    disp(c)
    disp(s_opt)
    disp(r_mu(:,:,j))
    % % % % % % % % % % % % % % % % % % % % % % % % % % % % % % % % % % % % % % % % % % % % % % % 

    % mu = mu./mu_decrease_rate;
    mu = mu/5;
    %mu(14:15) = mu(14:15)/25; 
end

Pb_bar = Pb_fun(x_bar(:,1),u_bar(:,1),du(:,1));
u1    = u_bar(:,1) + du(:,1); 
u_bar = u_bar + du;
x_bar_next = x_opt(:,2);


nominal.u_b = u_bar;
nominal.du = du;
nominal.du_IP = du_IP;
nominal.K0 = K0;
nominal.K0_IP = K0_IP;
nominal.x_opt = x_opt;
nominal.x_opt_IP = x_opt_IP;

nominal_IP_Bus.u_b = u_bar;
nominal_IP_Bus.du = du;
nominal_IP_Bus.K0 = K0;
nominal_IP_Bus.x_opt = x_opt;
nominal_IP_Bus.s = s_opt;

== matlab function main_ddp_N5/IP_ILQR_controller_test/AL-ILQR1 ==
  data: x input size=params.nx; u_bar input size=[params.nu,params.MPC.N]; du1 output size=params.nu; Pd input; K0 output size=[params.nu,params.nx]; u_bar output size=[params.nu,params.MPC.N]; params parameter; x_ output size=params.nx; Ref parameter; Smax input; u_b input; u_b output; ub1 output size=[params.nu 1]; Pb_bar output size=1; rammda input; rammda output; time_ILQR output size=1
function [du1,K0,u_bar,x_,u_b,ub1,Pb_bar,rammda,time_ILQR] = solve_snapshot(x,u_bar,Pd,params,Ref,Smax,u_b,rammda)
% One fixed OCP. This same source is installed in the two Simulink charts.
N = 5;
du=u_bar-u_b; nc=15;
K0=zeros(3,8); X=zeros(8,N+1);
Altro.mu=repmat(4e-4,nc,N+1);
Altro.I_mu=zeros(nc,nc*(N+1));
Altro.rammda=zeros(nc,N+1);
Altro.cmax=1e-8; Altro.phi=2;
C=ones(nc,N+1);
t0=tic;
for iter=1:params.N_iter
    for k=1:N+1
        for j=1:nc
            if C(j,k)<0 && Altro.rammda(j,k)==0
                Altro.I_mu(j,nc*(k-1)+j)=0;
            else
                Altro.I_mu(j,nc*(k-1)+j)=Altro.mu(j,k);
            end
        end
    end
    [X,A,B]=forwardpass_exp(x,u_b,du,params.tsp_str,N,params,Ref);
    [du,K0,X]=backwardpass_exp(X,u_b,du,A,B,N,params.J_tsp,params.tsp_str, ...
        1,Pd,params,Altro,Ref,Smax,u_b);
    for k=1:N+1
        j=min(k,N);
        if (X(1,k)/.1173+params.psat/Ref.pres)<2
            C(:,k)=constraints_case1(X(:,k),u_b(:,j),du(:,j),Pd(k),Smax);
        else
            C(:,k)=constraints_case2(X(:,k),u_b(:,j),du(:,j),Pd(k),Smax);
        end
        % All 15 constraints are inequalities. Update on violations as well.
        Altro.rammda(:,k)=max(0,Altro.rammda(:,k)+Altro.mu(:,k).*C(:,k));
        for j=1:nc
            if C(j,k)>1e-6
                Altro.mu(j,k)=min(100,2*Altro.mu(j,k));
            end
        end
    end
end
rammda=circshift(Altro.rammda,-1,2); rammda(:,end)=rammda(:,end-1);
x_=X(:,2); du1=du(:,1); ub1=u_b(:,1);
Pb_bar=Pb_fun(X(:,1),u_b(:,1),du(:,1));
u_b=u_b+du; u_bar=[u_b(:,2:end),u_b(:,end)];
if isfield(params,'closed_loop_feedback') && params.closed_loop_feedback==0
    K0(:)=0; % same intersample policy as the fmincon reference
end
time_ILQR=toc(t0);
end

== matlab function main_ddp_N5/MATLAB Function7 ==
  data: x input; Ifc input; z output; params parameter
function z = fcn(x,Ifc,params)

z = params.c23*(x(4)-x(1)-x(2)-params.c2)/(params.c24*Ifc);

== matlab function main_ddp_N5/fuel_cel_systeml ==
  data: x input; Vcm input; Ifc input; Vfc output; Pcm output; params parameter
function [Vfc,Pcm] = fcn(x,Vcm,Ifc,params)
Pcm = Vcm*(Vcm-params.kv*x(3))/(params.Rcm*params.eata_cm);
Tfc = params.Tst;
po2 = x(1);
pH2 = x(1)+x(2);


E = 1.229-0.85e-3*(Tfc-params.Tatm)+4.3085e-5*Tfc*(reallog(pH2/params.patm)+1/2*reallog(po2/params.patm));
v0 = 0.279-8.5e-4*(Tfc-params.Tatm)+4.308e-5*Tfc*(reallog((x(1)+x(2))/params.patm)+1/2*reallog(0.1173*(x(1)+x(2))/params.patm));
va = (-1.68e-5*Tfc+1.618e-2)*(1.01325*(po2/0.1173+params.psat)/params.patm)^2+(1.8e-4*Tfc-0.166)*(1.01325*(po2/0.1173+params.psat)/params.patm)+(-5.8e-4*Tfc+0.5736);
a1 = 10;
I = Ifc/params.Afc;
vact = v0+va*(1-exp(-a1*I));
b11 = 5.139e-3;
b12 = 3.26e-3;
b2 = 350;
mu_m = 14; % vapor 100%
sig_m = (b11*mu_m-b12)*exp(b2*(1/303-1/Tfc));
Rohm = params.tm/sig_m;
vohm = I*Rohm;

if (po2/0.1173+params.psat) < 2*params.patm
a2 = (7.16e-4*Tfc-0.622)*1.01325*(po2/0.1173+params.psat)/params.patm+(-1.45e-3*Tfc+1.68);
else 
a2 = (8.66e-5*Tfc-0.068)*1.01325*(po2/0.1173+params.psat)/params.patm+(-1.6e-4*Tfc+0.54);
end
Imax = 2.2;
a3 = 2;
vconc = I*(a2*I/Imax)^a3;

vfc = E-vact-vohm-vconc;
Vfc = vfc*params.n;

== matlab function main_ddp_N5/MATLAB Function ==
  data: Batt input; Pb output; Ib input; Vb output; params parameter
function [Pb,Vb] = fcn(Batt,Ib,params)
% Ib = Ib/15; %pararel
Ib = Ib/params.battery.parallel; %pararel
Vsoc = Batt(1);
Vs = Batt(2);
Vf = Batt(3);
SOC = Vsoc ;
Voc = -1.031*exp(-35*SOC)+3.685+0.2156*SOC-0.1178*SOC^2+0.3201*SOC^3;
R0 = 0.1562*exp(-24.37*SOC)+0.07446;
Vb = Voc-R0*Ib-Vs-Vf;
% Ib = Ib*15;
Ib = Ib*params.battery.parallel;
Vb = Vb*params.battery.series;
% Pb = Ib*Vb*12; %series 12
% Pb = Ib*Vb*params.battery.series; %series 12
Pb = Ib*Vb;

== matlab function main_ddp_N5/oldAL_ILQR_controller/MATLAB QDDP1 ==
  data: x input size=params.nx; u_bar input size=[params.nu,params.MPC.N]; du1 output size=params.nu; Pd input; K0 output size=[params.nu,params.nx]; u_bar output size=[params.nu,params.MPC.N]; params parameter; x_ output size=params.nx; Ref parameter; Smax input; u_b input; u_b output; ub1 output size=[params.nu 1]; Pb_bar output size=1; time input; rammda input; rammda output
function [du1,K0,u_bar,x_,u_b,ub1,Pb_bar,rammda] = QDDP(x,u_bar,Pd,params,Ref,Smax,u_b,time,rammda)
%UNTITLED3 この関数の概要をここに記述
%   詳細説明をここに記述
du = u_bar-u_b;
% whitch discretization method
D_method = 'V';     % D:difference, V:variational
if time >= 1.55
     disp(time)    
end
% x = x./[Ref.x;1;1;1];
% u_bar = u_bar./[Ref.Vcm;Ref.Ifc;Ref.Ib];
% linesearch off:0 on:1
linesearch = 1;
tsp = params.MPC.dt;  % sampling period
N = 10;      % number of horizon
N_iter = params.N_iter; % number of N_iter
% Max_N_iter_con = 100;

nx = size(x,1);
nu = size(u_bar,1);
K0 = zeros(nu,nx);
x_bar = zeros(nx,N+1);
x_bef = x_bar;
du_bef = u_bar;

lx = zeros(nx,N+1);
lu = zeros(nu,N);
Mxx = zeros(nx,(N+1)*nx);
Mux = zeros(nu,N*nx);
Muu = zeros(nu,N*nu);
A = zeros(nx,nx*N);
B = zeros(nx,nu*N);

nc = 15 ;
nc_i = params.nc_i;
% flag = true(nc,size(u_bar,2)+1);
Altro.mu = repmat(4e-4,nc,N+1);
% Altro.mu = repmat([1e-8;1e-2;1e-2;1e-8;1e-8;1e-8;1e-8;1e-8;1e-8;1e-8;1e-8;1e-8;1e-8;1e-8],N+1);
Altro.I_mu = zeros(nc,(N+1)*nc);
Altro.rammda = rammda;
% Altro.rammda = zeros(nc,N+1);
Altro.cmax = 1e-12;
Altro.phi = 2;
Value_c = ones(nc,N+1);
tolerance =1;
for i = 1:N_iter
    % for ii = 1:N+1
    %      for jj = 1:nc
    %             if Value_c(jj,ii) < 0 && Altro.rammda(jj,ii) == 0 && jj <= nc_i
    %                 Altro.I_mu(jj,nc*(ii-1)+jj) = 0;
    %             else
    %                 Altro.I_mu(jj,nc*(ii-1)+jj) = Altro.mu(jj,ii);
    %             end
    %             if Altro.mu(jj,ii)<=1e8
    %                 Altro.mu(jj,ii) = Altro.mu(jj,ii)*Altro.phi;
    %             end
    %      end
    % end
     for ii = 1:N+1
         for jj = 1:nc
                if Value_c(jj,ii) < 0 && Altro.rammda(jj,ii) == 0 && jj <= nc_i
                    Altro.I_mu(jj,nc*(ii-1)+jj) = 0;
                else
                    Altro.I_mu(jj,nc*(ii-1)+jj) = Altro.mu(jj,ii);
                if Altro.mu(jj,ii)<=100
                    Altro.mu(jj,ii) = Altro.mu(jj,ii)*Altro.phi;
                end
                end

         end
    end
     % if i == 44
          % disp(i)
          disp('--------------')
     % end
        A_bef = A;
        B_bef = B;

    [x_bar,A,B] = forwardpass(x,u_b,du,tsp,N,D_method,params,Ref);
        delta_x = x_bar-x_bef;
        delta_u = du-du_bef;
        du_bef = du;
    [du,K0,lx,lu,Mxx,Mux,Muu,x_bef,tolerance] = backwardpass_QDDP(x_bar,u_b,du,A,B,N,tsp,linesearch,Pd,params,Altro,Ref,Smax,u_b,lx,lu,delta_x,delta_u,Mxx,Mux,Muu,A_bef,B_bef);
    % [x_bar,A,B] = forwardpass_runge(x,u_b,du,tsp,N,D_method,params,Ref);
    % [du,K0] = backwardpass_Altro_e_runge(x_bar,u_b,du,A,B,N,tsp,linesearch,Pd,params,Altro,Ref,Smax);
        for ii = 1:N+1

            if ii ~= N+1
                [x_bar(:,ii),du(:,ii)] = satulation(x_bar(:,ii),u_b(:,ii),du(:,ii));
                if (x_bar(1,:)/0.1173+params.psat/Ref.pres) < 2
                    Value_c(:,ii) = constraints_case1(x_bar(:,ii),u_b(:,ii),du(:,ii),Pd(ii),Smax);
                else
                    Value_c(:,ii) = constraints_case2(x_bar(:,ii),u_b(:,ii),du(:,ii),Pd(ii),Smax);
                end
            else
                [x_bar(:,ii),~] = satulation(x_bar(:,ii),u_b(:,ii-1),du(:,ii-1));
                if (x_bar(1,:)/0.1173+params.psat/Ref.pres) < 2
                    Value_c(:,ii) = constraints_case1(x_bar(:,ii),u_b(:,ii-1),du(:,ii-1),Pd(ii-1),Smax);
                else
                    Value_c(:,ii) = constraints_case2(x_bar(:,ii),u_b(:,ii-1),du(:,ii-1),Pd(ii-1),Smax);
                end
            end

            % for jj = 1:nc
            % 
            %     if jj <=nc_i
            %         Altro.rammda(jj,ii) = max([Altro.rammda(jj,ii) + Altro.mu(jj,ii).*Value_c(jj,ii),0]);
            %     else
            %         Altro.rammda(jj,ii) = Altro.rammda(jj,ii) + Altro.mu(jj,ii).*Value_c(jj,ii);
            %     end
            % 
            % end
            for jj = 1:nc

                if Value_c(jj,ii) < 0 && Altro.rammda(jj,ii) == 0 && jj <= nc_i
                    Altro.rammda(jj,ii) = max([Altro.rammda(jj,ii) + Altro.mu(jj,ii).*Value_c(jj,ii),0]);
                elseif jj>nc_i
                    Altro.rammda(jj,ii) = Altro.rammda(jj,ii) + Altro.mu(jj,ii).*Value_c(jj,ii);
                else
                end

            end
            if all(abs(tolerance)<1e-8)
                if all(Value_c<=Altro.cmax)
                    disp(ii)
                    disp('o')
                    break
                end
            end
                    % disp(Altro.rammda(:,ii))
        end
end

rammda = circshift(Altro.rammda,-1,2);
% rammda(:,end) = zeros(nc,1);
ub1 = u_b(:,1);
u_bar = u_b+du;
% if any(Value_c(:,2)>0)
% disp(Value_c(:,2))
% disp('---------------------')
% end
Pb_bar = Pb_fun(x_bar(:,1),u_b(:,1),du(:,1));
x_ = x_bar(:,2);
du1 = du(:,1);
u_b = u_bar;
u_bar = circshift(u_b,-1,2);

u_bar(:,end) = u_b(:,end-1);



% function [du1,K0,u_bar,x_,u_b,ub1,Pb_bar] = ILQR(x,u_bar,Pd,params,Ref,Smax,u_b)
% %UNTITLED3 この関数の概要をここに記述
% %   詳細説明をここに記述
% % tic;
% du = u_bar-u_b;
% % whitch discretization method
% D_method = 'V';     % D:difference, V:variational
% % if time >= 2.4
% %      disp(time)    
% % end
% % x = x./[Ref.x;1;1;1];
% % u_bar = u_bar./[Ref.Vcm;Ref.Ifc;Ref.Ib];
% % linesearch off:0 on:1
% linesearch = 1;
% tsp = params.MPC.dt;  % sampling period
% N = 10;      % number of horizon
% N_iter = params.N_iter; % number of N_iter
% % Max_N_iter_con = 100;
% 
% nx = size(x,1);
% nu = size(u_bar,1);
% K0 = zeros(nu,nx);
% x_bar = zeros(nx,N+1);
% nc = 15 ;
% nc_i = params.nc_i;
% % flag = true(nc,size(u_bar,2)+1);
% Altro.mu = repmat(1e-6 ...
%     ,nc,N+1);
% % Altro.mu = repmat([1e-8;1e-2;1e-2;1e-8;1e-8;1e-8;1e-8;1e-8;1e-8;1e-8;1e-8;1e-8;1e-8;1e-8],N+1);
% Altro.I_mu = zeros(nc,(N+1)*nc);
% % Altro.rammda = rammda;
% Altro.rammda = zeros(nc,N+1);
% Altro.cmax = 1e-8;
% Altro.phi = 2;
% Value_c = ones(nc,N+1);
% 
% for i = 1:N_iter
%     % for ii = 1:N+1
%     %      for jj = 1:nc
%     %             if Value_c(jj,ii) < 0 && Altro.rammda(jj,ii) == 0 && jj <= nc_i
%     %                 Altro.I_mu(jj,nc*(ii-1)+jj) = 0;
%     %             else
%     %                 Altro.I_mu(jj,nc*(ii-1)+jj) = Altro.mu(jj,ii);
%     %             end
%     %             if Altro.mu(jj,ii)<=1e8
%     %                 Altro.mu(jj,ii) = Altro.mu(jj,ii)*Altro.phi;
%     %             end
%     %      end
%     % end
%      for ii = 1:N+1
%          for jj = 1:nc
%                 if Value_c(jj,ii) < 0 && Altro.rammda(jj,ii) == 0 && jj <= nc_i
%                     Altro.I_mu(jj,nc*(ii-1)+jj) = 0;
%                              %        else
%                     Altro.I_mu(jj,nc*(ii-1)+jj) = Altro.mu(jj,ii);
%                 if Altro.mu(jj,ii)<=100
%                     Altro.mu(jj,ii) = Altro.mu(jj,ii)*Altro.phi;
%                 end
%                 end
% 
%          end
%          %  for jj = 1:nc
%          %        if Value_c(jj,ii) < -Altro.rammda(jj,ii)/(2*Altro.mu(jj,ii)) && Altro.rammda(jj,ii) == 0 && jj <= nc_i
%          % 
%          %            Altro.I_mu(jj,nc*(ii-1)+jj) = 1/4*(Altro.rammda(jj,ii)^2/Altro.mu(jj,ii))/(Value_c(jj,ii)^2);
%          %        else
%          %            Altro.I_mu(jj,nc*(ii-1)+jj) = Altro.mu(jj,ii);
%          %        if Altro.mu(jj,ii)<=100
%          %            Altro.mu(jj,ii) = Altro.mu(jj,ii)*Altro.phi;
%          %        end
%          %        end
%          % 
%          % end
%     end
%      % if i == 44
%            disp(i)
%           % disp('--------------')
%      % end
%     [x_bar,A,B] = forwardpass(x,u_b,du,tsp,N,D_method,params,Ref);
%     [du,K0] = backwardpass_Altro_e(x_bar,u_b,du,A,B,N,tsp,linesearch,Pd,params,Altro,Ref,Smax);
%     % [x_bar,A,B] = forwardpass_runge(x,u_b,du,tsp,N,D_method,params,Ref);
%     % [du,K0] = backwardpass_Altro_e_runge(x_bar,u_b,du,A,B,N,tsp,linesearch,Pd,params,Altro,Ref,Smax);
% 
%         for ii = 1:N+1
% 
%             if ii ~= N+1
%                 [x_bar(:,ii),du(:,ii)] = satulation(x_bar(:,ii),u_b(:,ii),du(:,ii));
%                 if (x_bar(1,:)/0.1173+params.psat/Ref.pres) < 2
%                     Value_c(:,ii) = constraints_case1(x_bar(:,ii),u_b(:,ii),du(:,ii),Pd(ii),Smax);
%                 else
%                     Value_c(:,ii) = constraints_case2(x_bar(:,ii),u_b(:,ii),du(:,ii),Pd(ii),Smax);
%                 end
%             else
%                 [x_bar(:,ii),~] = satulation(x_bar(:,ii),u_b(:,ii-1),du(:,ii-1));
%                 if (x_bar(1,:)/0.1173+params.psat/Ref.pres) < 2
%                     Value_c(:,ii) = constraints_case1(x_bar(:,ii),u_b(:,ii-1),du(:,ii-1),Pd(ii-1),Smax);
%                 else
%                     Value_c(:,ii) = constraints_case2(x_bar(:,ii),u_b(:,ii-1),du(:,ii-1),Pd(ii-1),Smax);
%                 end
%             end
% 
%             % for jj = 1:nc
%             % 
%             %     if jj <=nc_i
%             %         Altro.rammda(jj,ii) = max([Altro.rammda(jj,ii) + Altro.mu(jj,ii).*Value_c(jj,ii),0]);
%             %     else
%             %         Altro.rammda(jj,ii) = Altro.rammda(jj,ii) + Altro.mu(jj,ii).*Value_c(jj,ii);
%             %     end
%             % 
%             % end
%             for jj = 1:nc
% 
%                 if Value_c(jj,ii) < 0 && Altro.rammda(jj,ii) == 0 && jj <= nc_i
%                     Altro.rammda(jj,ii) = max([Altro.rammda(jj,ii) + Altro.mu(jj,ii).*Value_c(jj,ii),0]);
%                 elseif jj>nc_i
%                     Altro.rammda(jj,ii) = Altro.rammda(jj,ii) + Altro.mu(jj,ii).*Value_c(jj,ii);
%                 else
%                 % if Value_c(jj,ii) < -Altro.rammda(jj,ii)/(2*Altro.mu(jj,ii)) && Altro.rammda(jj,ii) == 0 && jj <= nc_i
%                 %     Altro.rammda(jj,ii) = max([Altro.rammda(jj,ii) + Altro.mu(jj,ii).*Value_c(jj,ii),-1/4*(Altro.rammda(jj,ii)^2/Altro.mu(jj,ii))/(Value_c(jj,ii))]);
%                 % elseif jj>nc_i
%                 %     Altro.rammda(jj,ii) = Altro.rammda(jj,ii) + Altro.mu(jj,ii).*Value_c(jj,ii);
%                 % else
% 
%                 end
% 
%             end
%             % disp(Altro.rammda(:,ii))
%         end
% end
% % rammda = circshift(Altro.rammda,-1,2);
% % rammda(:,end) = rammda(:,end-1);
% ub1 = u_b(:,1);
% u_bar = u_b+du;
% % if any(Value_c(:,2)>0)
% % disp(Value_c(:,2))
% % disp('---------------------')
% % end
% Pb_bar = Pb_fun(x_bar(:,1),u_b(:,1),du(:,1));
% x_ = x_bar(:,2);
% du1 = du(:,1);
% u_b = u_bar;
% u_bar = circshift(u_b,-1,2);
% % disp(toc)
% u_bar(:,end) = u_b(:,end-1);
